simulink model "sens_mtr"  (R2022a)
settings: Solver=FixedStepAuto  StartTime=0.0  StopTime=10.0  RelTol=1e-3  EnableMultiTasking=on
libraries: mbedblockslib x9, hdlsllib x1
settings Model: ExtModeTrigDuration=10  Creator=MATLAB  LastModifiedBy=MATLAB
settings OptimizationCC: EnhancedBackFolding=on  PassReuseOutputArgsAs=Individual arguments  ZeroExternalMemoryAtStartup=off  ZeroInternalMemoryAtStartup=off  MaxStackSize=64  OptimizeBlockOrder=speed  DifferentSizesBufferReuse=on  OptimizationCustomize=off  EfficientTunableParamExpr=on
settings DebuggingCC: ParameterTunabilityLossMsg=error  UnconnectedInputMsg=warning  UnconnectedOutputMsg=warning  UnconnectedLineMsg=warning
settings HardwareCC: ProdBitPerPointer=32  ProdBitPerSizeT=32  ProdBitPerPtrDiffT=32  ProdLargestAtomicInteger=Long  ProdLargestAtomicFloat=Double  ProdWordSize=32  ProdHWDeviceType=ARM Compatible->ARM Cortex
settings SFSimCC: MATLABDynamicMemAlloc=off
settings RTWCC: SystemTargetFile=ert.tlc  HardwareBoard=STM32 Nucleo L476RG  TemplateMakefile=ert_default_tmf  Toolchain=GNU Tools for ARM Embedded Processors  DLArmComputeVersion=19.05
settings CodeAppCC: ForceParamTrailComments=on  IgnoreCustomStorageClasses=off  OperatorAnnotations=on  SimulinkDataObjDesc=on  SFDataObjDesc=on  InsertBlockDesc=on
settings ERTTargetCC: ExtModeTransport=3  ExtModeStaticAlloc=on  ExtModeStaticAllocSize=2000  ExtModeMexFile=ext_xcp  ExtModeIntrfLevel=Level2 - Open

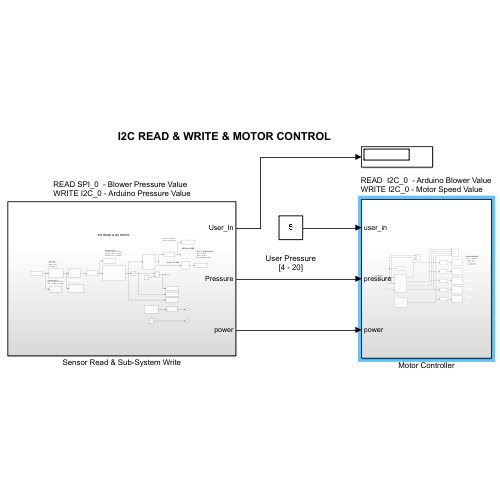
[thumbnail: Simulink's stored preview of the top-level diagram]
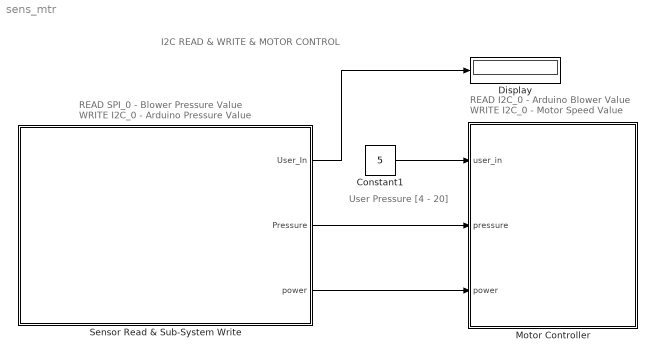
== system sens_mtr ==
  note: User Pressure
      | [4 - 20]
  note: READ SPI_0  - Blower Pressure Value
      | WRITE I2C_0 - Arduino Pressure Value
  note: I2C READ & WRITE & MOTOR CONTROL
  note: READ  I2C_0  - Arduino Blower Value
      | WRITE I2C_0 - Motor Speed Value
  Constant1 : Constant  Value=5
  Display : Display
  Motor Controller : Subsystem
  Sensor Read & Sub-System Write : Subsystem
  wires:
  Sensor Read & Sub-System Write/3(power) -> Motor Controller/3(power)
  Sensor Read & Sub-System Write/2(Pressure) -> Motor Controller/2(pressure)
  Sensor Read & Sub-System Write/1(User_In) -> Display/1
  Constant1/1 -> Motor Controller/1(user_in)

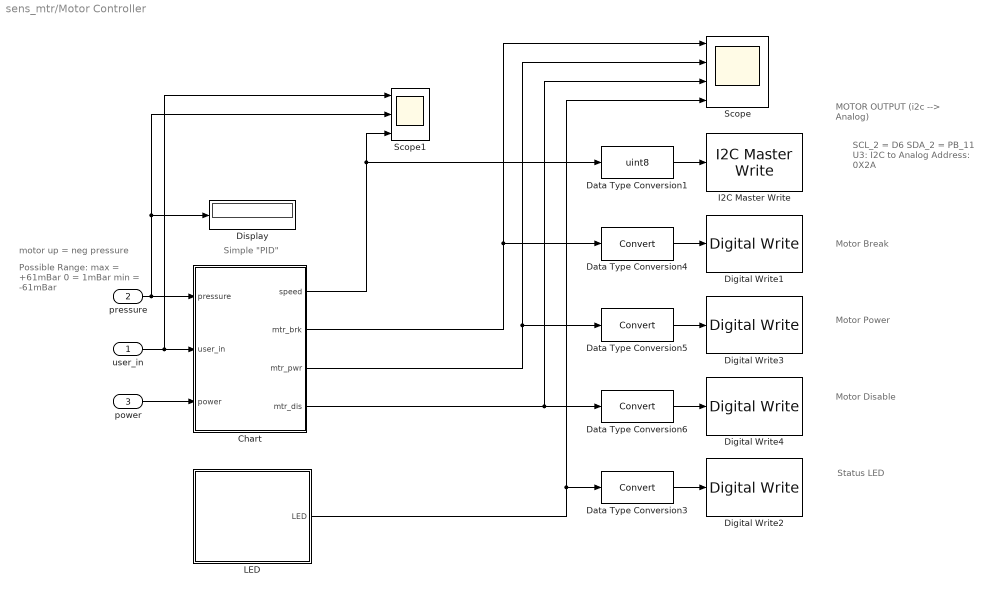
== system sens_mtr/Motor Controller ==
  note: motor up = neg pressure
  note: MOTOR OUTPUT
      | (i2c --> Analog)
  note: SCL_2 = D6
      | SDA_2 = PB_11
      | U3: I2C to Analog
      | Address: 0X2A
  note: Motor Break
  note: Motor Power
  note: Motor Disable
  note: Simple "PID"
  note: Possible Range:
      | max = +61mBar
      | 0 = 1mBar
      | min = -61mBar
  note: Status LED
  user_in : Inport
  pressure : Inport  Port=2
  power : Inport  Port=3
  Chart : Stateflow chart  TreatAsAtomicUnit=on
  Data Type Conversion1 : DataTypeConversion  OutDataTypeStr=uint8  SaturateOnIntegerOverflow=off  RndMeth=Floor
  Data Type Conversion{3..6} (4 alike) : DataTypeConversion  SaturateOnIntegerOverflow=off  RndMeth=Floor
  Digital Write1 : mbedblockslib/Digital Write  Pin=PC_3  Direction=output
      settings: SourceProductBaseCode=MICROBIT,NUCLEO,STMICRODIS
  Digital Write2 : mbedblockslib/Digital Write  Pin=PB_0  Direction=output
      settings: SourceProductBaseCode=MICROBIT,NUCLEO,STMICRODIS
  Digital Write3 : mbedblockslib/Digital Write  Pin=PB_9  Direction=output
      settings: SourceProductBaseCode=MICROBIT,NUCLEO,STMICRODIS
  Digital Write4 : mbedblockslib/Digital Write  Pin=PC_4  Direction=output
      settings: SourceProductBaseCode=MICROBIT,NUCLEO,STMICRODIS
  Display : Display
  I2C Master Write : mbedblockslib/I2C Master Write  I2CModule=2  Mode=Master  SlaveAddress=uint8(hex2dec('2A'))  SlaveByteOrder=BigEndian  Direction=Transmitter  RegisterAddressMode=on  RegisterAddress=uint8(hex2dec('10'))  SlaveDataType=uint8  DataLength=2  NoAck=off  RepeatedStart=off  OutputStatus=off
      settings: SourceProductBaseCode=MICROBIT,NUCLEO,STMICRODIS
  LED : Stateflow chart  TreatAsAtomicUnit=on
  Scope : Scope  NumInputPorts=4
  Scope1 : Scope  NumInputPorts=3
  wires:
  Data Type Conversion1/1 -> I2C Master Write/1
  Data Type Conversion5/1 -> Digital Write3/1
  Chart/2(mtr_brk) -> Data Type Conversion4/1, Scope/1
  Chart/4(mtr_dis) -> Data Type Conversion6/1, Scope/3
  Chart/1(speed) -> Data Type Conversion1/1, Scope1/3
  Data Type Conversion4/1 -> Digital Write1/1
  Chart/3(mtr_pwr) -> Scope/2, Data Type Conversion5/1
  Data Type Conversion6/1 -> Digital Write4/1
  pressure/1 -> Display/1, Scope1/2, Chart/1(pressure)
  user_in/1 -> Scope1/1, Chart/2(user_in)
  power/1 -> Chart/3(power)
  Data Type Conversion3/1 -> Digital Write2/1
  LED/1(LED) -> Scope/4, Data Type Conversion3/1

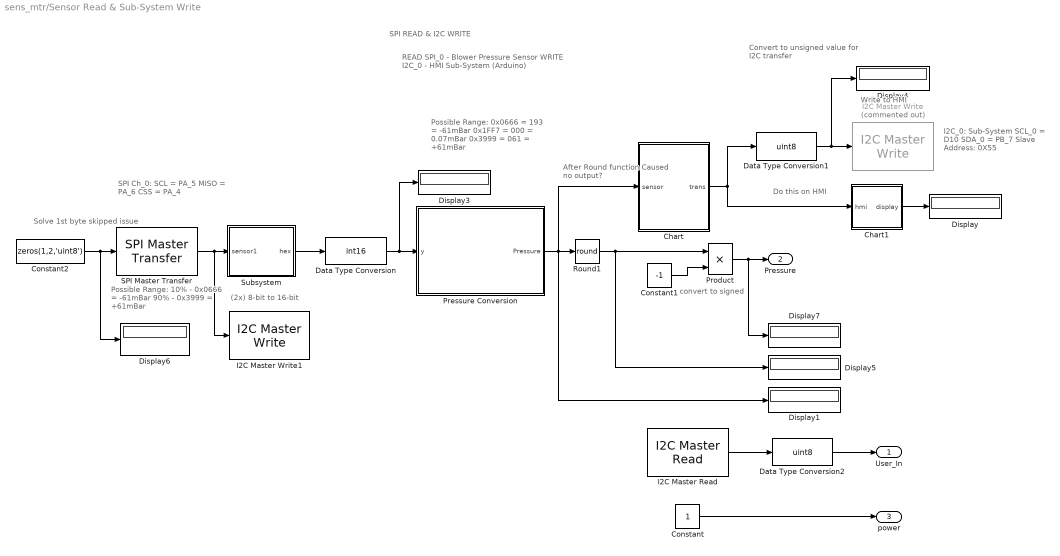
== system sens_mtr/Sensor Read & Sub-System Write ==
  note: After Round function
      | Caused no output?
  note: convert to signed
  note: (2x) 8-bit to 16-bit
  note: SPI READ & I2C WRITE
  note: READ SPI_0  -  Blower Pressure Sensor
      | WRITE I2C_0 - HMI Sub-System (Arduino)
  note: SPI Ch_0:
      | SCL = PA_5
      | MISO = PA_6
      | CSS = PA_4
  note: I2C_0: Sub-System
      | SCL_0 = D10
      | SDA_0 = PB_7
      | Slave Address: 0X55
  note: Possible Range:
      | 10% - 0x0666 = -61mBar
      | 90% - 0x3999 = +61mBar
  note: Possible Range:
      | 0x0666 = 193 = -61mBar
      | 0x1FF7 = 000 = 0.07mBar
      | 0x3999 = 061 = +61mBar
  note: Write to HMI
  note: Do this on HMI
  note: Convert to unsigned
      | value for I2C transfer
  note: Solve 1st byte
      | skipped issue
  Chart : Stateflow chart  TreatAsAtomicUnit=on
  Chart1 : Stateflow chart  TreatAsAtomicUnit=on
  Constant : Constant
  Constant1 : Constant  Value=-1
  Constant2 : Constant  Value=zeros(1,2,'uint8')  OutDataTypeStr=uint8
  Data Type Conversion : DataTypeConversion  OutDataTypeStr=int16  SaturateOnIntegerOverflow=off  RndMeth=Floor
  Data Type Conversion1 : DataTypeConversion  OutDataTypeStr=uint8  SaturateOnIntegerOverflow=off  RndMeth=Floor
  Data Type Conversion2 : DataTypeConversion  OutDataTypeStr=uint8  SaturateOnIntegerOverflow=off  RndMeth=Floor
  Display{,1,3..7} (7 alike) : Display
      Display3 settings: Format=hex (Stored Integer)
      Display6 settings: Format=hex (Stored Integer)
  I2C Master Read : mbedblockslib/I2C Master Read  I2CModule=0  Mode=Master  SlaveAddress=hex2dec('55')  SlaveByteOrder=BigEndian  Direction=Receiver  RegisterAddressMode=off  RegisterAddress=uint8(1)  SlaveDataType=uint8  DataLength=1  NoAck=off  RepeatedStart=off  OutputStatus=off  SampleTime=0.1
      settings: SourceProductBaseCode=MICROBIT,NUCLEO,STMICRODIS
  I2C Master Write : mbedblockslib/I2C Master Write  Commented=on  I2CModule=0  Mode=Master  SlaveAddress=uint8(hex2dec('55'))  SlaveByteOrder=BigEndian  Direction=Transmitter  RegisterAddressMode=off  RegisterAddress=uint8(hex2dec('11'))  SlaveDataType=uint8  DataLength=2  NoAck=off  RepeatedStart=off  OutputStatus=off
      settings: SourceProductBaseCode=MICROBIT,NUCLEO,STMICRODIS
  I2C Master Write1 : mbedblockslib/I2C Master Write  I2CModule=0  Mode=Master  SlaveAddress=uint8(hex2dec('55'))  SlaveByteOrder=BigEndian  Direction=Transmitter  RegisterAddressMode=off  RegisterAddress=uint8(hex2dec('11'))  SlaveDataType=uint8  DataLength=2  NoAck=off  RepeatedStart=off  OutputStatus=off
      settings: SourceProductBaseCode=MICROBIT,NUCLEO,STMICRODIS
  Pressure Conversion : Subsystem
  Product : Product
  Round1 : Rounding  Operator=round
  SPI Master Transfer : mbedblockslib/SPI Master Transfer  SPIModule=0  Mode=Master  BusSpeed=uint32( 1000000 )  Pin=PA_4  FirstBitToTransfer=Most significant bit (MSB)  ClockMode=0  BlockFunction=Transfer  RegisterAddress=0  OutputDataType=int8  OutputDataLength=1  UseCustomSSPin=Explicit GPIO calls  ActiveLowSSPin=Active low
      settings: SourceProductBaseCode=MICROBIT,NUCLEO,STMICRODIS
  Subsystem : Subsystem
  User_In : Outport
  Pressure : Outport  Port=2
  power : Outport  Port=3
  wires:
  SPI Master Transfer/1 -> I2C Master Write1/1, Subsystem/1(sensor1)
  Subsystem/1(hex) -> Data Type Conversion/1
  Data Type Conversion/1 -> Display3/1, Pressure Conversion/1(y)
  Pressure Conversion/1(Pressure) -> Chart/1(sensor), Display1/1, Round1/1
  Constant2/1 -> Display6/1, SPI Master Transfer/1
  Chart1/1(display) -> Display/1
  Data Type Conversion1/1 -> I2C Master Write/1, Display4/1
  Chart/1(trans) -> Chart1/1(hmi), Data Type Conversion1/1
  Round1/1 -> Product/1, Display5/1
  Product/1 -> Display7/1, Pressure/1
  Constant1/1 -> Product/2
  I2C Master Read/1 -> Data Type Conversion2/1
  Data Type Conversion2/1 -> User_In/1
  Constant/1 -> power/1

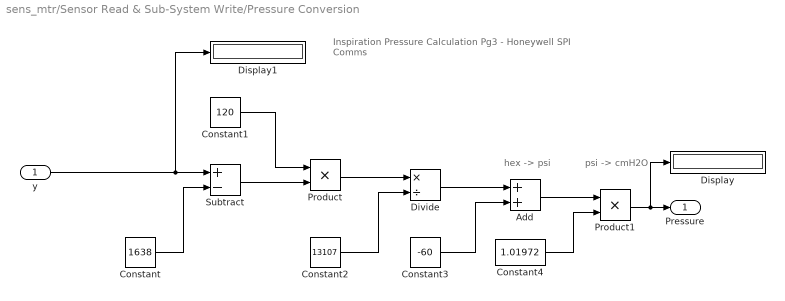
== system sens_mtr/Sensor Read & Sub-System Write/Pressure Conversion ==
  note: psi -> cmH2O
  note: Inspiration Pressure Calculation
      | Pg3 - Honeywell SPI Comms
  note: hex -> psi
  y : Inport
  Add : Sum
  Constant : Constant  Value=1638
  Constant1 : Constant  Value=120
  Constant2 : Constant  Value=13107
  Constant3 : Constant  Value=-60
  Constant4 : Constant  Value=1.01972
  Display : Display
  Display1 : Display
      settings: Format=hex (Stored Integer)
  Divide : Product  Inputs=*/
  Product : Product
  Product1 : Product
  Subtract : Sum  Inputs=+-
  Pressure : Outport
  wires:
  Constant/1 -> Subtract/2
  Subtract/1 -> Product/2
  Constant1/1 -> Product/1
  Product/1 -> Divide/1
  Constant2/1 -> Divide/2
  Constant3/1 -> Add/2
  Divide/1 -> Add/1
  Add/1 -> Product1/1
  Constant4/1 -> Product1/2
  Product1/1 -> Display/1, Pressure/1
  y/1 -> Display1/1, Subtract/1

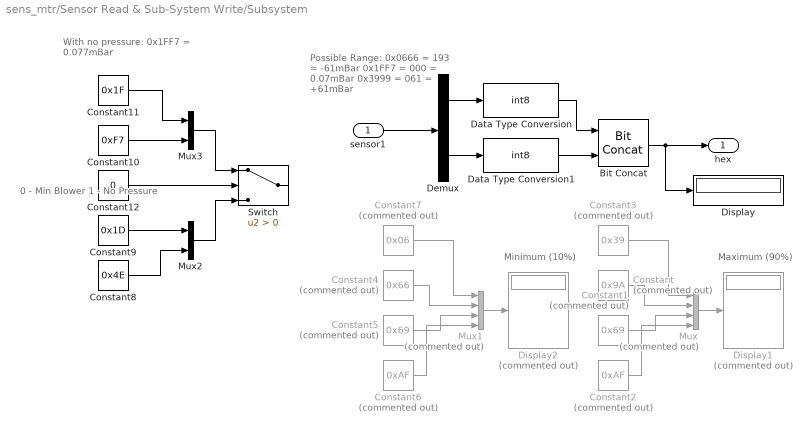
== system sens_mtr/Sensor Read & Sub-System Write/Subsystem ==
  note: 0 - Min Blower
      | 1 - No Pressure
  note: With no pressure:
      | 0x1FF7 = 0.077mBar
  note: Maximum (90%)
  note: Minimum (10%)
  note: Possible Range:
      | 0x0666 = 193 = -61mBar
      | 0x1FF7 = 000 = 0.07mBar
      | 0x3999 = 061 = +61mBar
  sensor1 : Inport
  Bit Concat : hdlsllib/Logic and Bit Operations/Bit Concat  numInputs=2
  Constant : Constant  Commented=on  Value=0x9A
  Constant1 : Constant  Commented=on  Value=0x69
  Constant10 : Constant  Value=0xF7
  Constant11 : Constant  Value=0x1F
  Constant12 : Constant  Value=0
  Constant2 : Constant  Commented=on  Value=0xAF
  Constant3 : Constant  Commented=on  Value=0x39
  Constant4 : Constant  Commented=on  Value=0x66
  Constant5 : Constant  Commented=on  Value=0x69
  Constant6 : Constant  Commented=on  Value=0xAF
  Constant7 : Constant  Commented=on  Value=0x06
  Constant8 : Constant  Value=0x4E
  Constant9 : Constant  Value=0x1D
  Data Type Conversion : DataTypeConversion  OutDataTypeStr=int8  SaturateOnIntegerOverflow=off  RndMeth=Floor
  Data Type Conversion1 : DataTypeConversion  OutDataTypeStr=int8  SaturateOnIntegerOverflow=off  RndMeth=Floor
  Demux : Demux  Outputs=2
  Display : Display
      settings: Format=hex (Stored Integer)
  Display1 : Display  Commented=on
      settings: Format=hex (Stored Integer)
  Display2 : Display  Commented=on
      settings: Format=hex (Stored Integer)
  Mux : Mux  Commented=on
  Mux1 : Mux  Commented=on
  Mux2 : Mux  Inputs=2
  Mux3 : Mux  Inputs=2
  Switch : Switch  Criteria=u2 > Threshold  SaturateOnIntegerOverflow=off  InputSameDT=off
  hex : Outport
  wires:
  Constant3/1 -> Mux/1
  Constant/1 -> Mux/2
  Constant1/1 -> Mux/3
  Constant2/1 -> Mux/4
  Data Type Conversion/1 -> Bit Concat/1
  Data Type Conversion1/1 -> Bit Concat/2
  Demux/1 -> Data Type Conversion/1
  Demux/2 -> Data Type Conversion1/1
  Bit Concat/1 -> hex/1, Display/1
  Mux/1 -> Display1/1
  Mux1/1 -> Display2/1
  Constant7/1 -> Mux1/1
  Constant6/1 -> Mux1/4
  Constant5/1 -> Mux1/3
  Constant4/1 -> Mux1/2
  Constant9/1 -> Mux2/1
  Constant8/1 -> Mux2/2
  Constant10/1 -> Mux3/2
  Constant11/1 -> Mux3/1
  Constant12/1 -> Switch/2
  Mux3/1 -> Switch/1
  Mux2/1 -> Switch/3
  sensor1/1 -> Demux/1

== stateflow chart sens_mtr/Motor Controller/LED ==
  note: TEST:
      | Routine Checks
  state Run % Parent
    state Check % Check Sub-Systems
      entry:
      LED = 0; % LED Off
      exit:
    state LED % Child
      entry: % none
      LED = 1; % LED On
      exit: % none
    (default) -> LED % Child
    LED % Child -> Check % Check Sub-Systems : after(2,sec)
    Check % Check Sub-Systems -> LED % Child : after(2,sec)
  note: Check Input
      | Power present?
  (default) -> Run % Parent
  data: LED output

== stateflow chart sens_mtr/Motor Controller/Chart ==
  state MOTOR
    note: Unused for now...
    note: Adjust according to User Value?
    state SHUTDOWN % Blower Off
      state Stop_1 % I2C to Anal.
        entry:
        speed = 0x00; % slowest?
        %LED = 1;
        exit:
      state Stop_2 % Motor Brake
        entry:
        mtr_brk = 0; % Enable
        %LED = 0; % debug
        exit:
      state Stop_3 % Motor Disable
        entry:
        mtr_dis = 0; % Disable
        %LED = 1; % debug
        exit:
      state Stop_4 % Main Power
        entry:
        mtr_pwr = 0; % OFF
        % LED = 0; % debug
        exit:
      (default) -> Stop_1 % I2C to Anal.
      Stop_1 % I2C to Anal. -> Stop_2 % Motor Brake : after(2,sec)
      Stop_2 % Motor Brake -> Stop_3 % Motor Disable : after(2,sec)
      Stop_3 % Motor Disable -> Stop_4 % Main Power : after(2,sec)
    state STARTUP % Blower Start
      state Start_1 % Main Power
        entry:
        mtr_pwr = 1; % ON
        %LED = 1; % debug
        exit:
      state Start_2 % Motor Brake
        entry:
        mtr_brk = 1; % Disable
        mtr_dis = 1; % Enabled
        %LED = 0; % debug
        exit:
      (default) -> Start_1 % Main Power
      Start_1 % Main Power -> Start_2 % Motor Brake : after(1,sec)
    state PID % Adjust 10 time per sec?
      note: User Range:
          | max = 20
          | min = 4
      state PID_1
        entry: temp = 10;
        % Start in the middle
        speed = temp;
        exit:
      note: Speed Values:
          | 0xA0 = 3/4 Vout
          | 0x80 = 1/2 Vout
          | 0x40 = 1/4 Vout
      note: Pressure Range:
          | max = +61mBar
          | 0 = 1mBar
          | min = -61mBar
      state PID_2
        entry:
        % slow value follwer
        speed = temp;
        exit:
      state Decrement1
        entry:
        if(speed > 10)
        temp = speed - 5;
        end
        exit:
      state Increment
        entry:
        if(speed < 250)
        temp = speed + 5;
        end
        exit:
      (default) -> PID_1
      PID_1 -> PID_2 : after(100,msec)
      Decrement1 -> PID_2 : after(50,msec)
      Increment -> PID_2 : after(50,msec)
      PID_2 -> (junction 67)
      (junction 67) -> (junction 69)
      (junction 69) -> Increment [order 1] : [pressure < user_in]
      (junction 69) -> Decrement1 [order 2] : [pressure > user_in]
    note: 1. Power - On
        | 2. Brake - Off
        | 3. Disable - Off
        | 4. Voltage Output
    note: BRAKE PIN:
        | Enabled = <0.8V or Gnd
        | Deactivated = >2.4V or Not wired
    note: DISABLE PIN:
        | Disable = <0.8V or Gnd
        | Enable = >2.4V or Not wired
    note: "speed" must increase/decrease until "pressure" = "user_in"
    note: Compensate for negative pressures (-61 -> 0)
    note: NOTE:
        | * Large step sizes - Shift values faster
        | * Small step sizes - Closer to required value
    (default) -> STARTUP % Blower Start
    STARTUP % Blower Start -> PID % Adjust 10 time per sec? : after(2,sec)
    PID % Adjust 10 time per sec? -> SHUTDOWN % Blower Off : after(120, sec)
  (default) -> MOTOR
  data: speed output; mtr_brk output; mtr_pwr output; mtr_dis output; pressure input; user_in input; power input; temp local uint8

== stateflow chart sens_mtr/Sensor Read & Sub-System Write/Chart1 ==
  state entry_
    if(hmi < 62)
    display = hmi;
    else % Positive-Negative
    display = hmi - 255;
    end
  (default) -> entry_
  data: hmi input; display output

== stateflow chart sens_mtr/Sensor Read & Sub-System Write/Chart ==
  state Pos_Neg
    entry:
    if(sensor >= 0)
    trans = sensor;
    %elseif(sensor == -0)
    %   trans = 1;
    else % negative to Positive
    trans = 255 + sensor;
    end
  (default) -> Pos_Neg
  data: sensor input; trans output
